simulink model "Verification"  (R2012b)
settings: Solver=FixedStepDiscrete  StartTime=0.0  StopTime=500  FixedStep=0.1  RelTol=1e-3
values from neighbouring files (symbols this model uses):
  high_safety_margin_s = 3.0    (= 3)    [constants.m]
  low_safety_margin_s = 3.0    (= 3)    [constants.m]
  tank1_cross_section_area_m2 = 1    [constants.m]
  tank1_max_vol_m3 = 7    [constants.m]
  tank1_safety_hi_ht_m = 5.0    (= 5)    [constants.m]
  tank1_safety_lo_ht_m = 2.0    (= 2)    [constants.m]
  tank2_cross_section_area_m2 = 2    [constants.m]
  tank2_max_vol_m3 = 8    [constants.m]
  tank2_safety_hi_ht_m = 3.0    (= 3)    [constants.m]
  time_increment_s = 0.1    [constants.m]
libraries: sldvlib x8
settings Model: Creator=Kerianne  LastModifiedBy=Kerianne
settings OptimizationCC: InlineParams=on

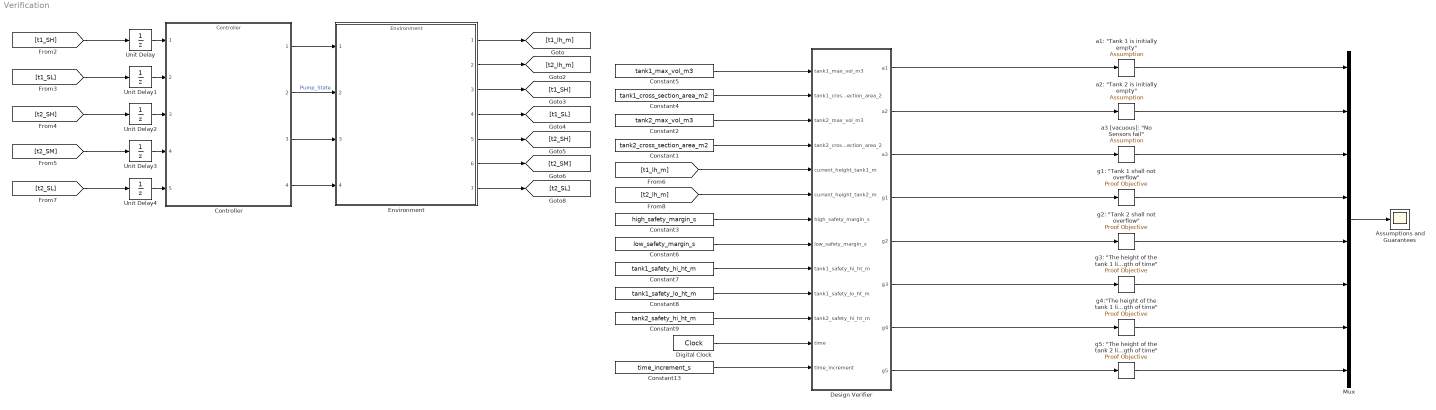
== system Verification ==
  " a2: \"Tank 2 is initially empty\" " : sldvlib/Objectives and Constraints/Assumption  enabled=on  customAVTBlockType=Assumption  intervals=true  initial=off  dispValues=on  outEnabled=on
      settings: AttributesFormatString=%<intervals>
  Assumptions and Guarantees : Scope
      settings: ShowLegends=on  TimeRange=500  YMin=0  YMax=2
  Constant1 : Constant  Value=tank2_cross_section_area_m2
  Constant13 : Constant  Value=time_increment_s
  Constant2 : Constant  Value=tank2_max_vol_m3
  Constant3 : Constant  Value=high_safety_margin_s
  Constant4 : Constant  Value=tank1_cross_section_area_m2
  Constant5 : Constant  Value=tank1_max_vol_m3
  Constant6 : Constant  Value=low_safety_margin_s
  Constant7 : Constant  Value=tank1_safety_hi_ht_m
  Constant8 : Constant  Value=tank1_safety_lo_ht_m
  Constant9 : Constant  Value=tank2_safety_hi_ht_m
  Controller : ModelReference  ModelNameDialog=Controller  SimulationMode=Normal  ModelReferenceVersion=1.19  CopyOfModelName=Controller  DefaultDataLogging=on
  Design Verifier : MATLAB Function  TreatAsAtomicUnit=on
  Digital Clock : DigitalClock  SampleTime=0.1
  Environment : ModelReference  ModelNameDialog=Environment  SimulationMode=Normal  ModelReferenceVersion=1.47  CopyOfModelName=Environment  DefaultDataLogging=on
  Mux : Mux  Inputs=8
  Unit Delay{,1..4} (5 alike) : UnitDelay  SampleTime=-1
  "a1: \"Tank 1 is initially empty\" " : sldvlib/Objectives and Constraints/Assumption  enabled=on  customAVTBlockType=Assumption  intervals=true  initial=off  dispValues=on  outEnabled=on
      settings: AttributesFormatString=%<intervals>
  "a3 [vacuous]: \"No Sensors fail\" " : sldvlib/Objectives and Constraints/Assumption  enabled=on  customAVTBlockType=Assumption  intervals=true  initial=off  dispValues=on  outEnabled=on
      settings: AttributesFormatString=%<intervals>
  "g1: \"Tank 1 shall not overflow\"" : sldvlib/Objectives and Constraints/Proof Objective  enabled=on  customAVTBlockType=Proof Objective  intervals=true  dispValues=on  outEnabled=on  enableStopSim=off
      settings: AttributesFormatString=%<intervals>
  "g2: \"Tank 2 shall not overflow\"" : sldvlib/Objectives and Constraints/Proof Objective  enabled=on  customAVTBlockType=Proof Objective  intervals=true  dispValues=on  outEnabled=on  enableStopSim=off
      settings: AttributesFormatString=%<intervals>
  "g3: \"The height of the tank 1 liquid shall not be over the tank 1 high safety level for more than the specified length of time\"" : sldvlib/Objectives and Constraints/Proof Objective  enabled=on  customAVTBlockType=Proof Objective  intervals=true  dispValues=on  outEnabled=on  enableStopSim=off
      settings: AttributesFormatString=%<intervals>
  "g4:\"The height of the tank 1 liquid shall not be lower than the tank 1 low safety level (once it has already crossed it) for more than the specified length of time\"" : sldvlib/Objectives and Constraints/Proof Objective  enabled=on  customAVTBlockType=Proof Objective  intervals=true  dispValues=on  outEnabled=on  enableStopSim=off
      settings: AttributesFormatString=%<intervals>
  "g5: \"The height of the tank 2 liquid shall not be over the tank 2 high safety level for more than the specified length of time\"" : sldvlib/Objectives and Constraints/Proof Objective  enabled=on  customAVTBlockType=Proof Objective  intervals=true  dispValues=on  outEnabled=on  enableStopSim=off
      settings: AttributesFormatString=%<intervals>
  wires:
  Design Verifier/1(a1) -> "a1: \"Tank 1 is initially empty\" "/1
  Digital Clock/1 -> Design Verifier/12(time)
  [t1_lh_m] -> Design Verifier/5(current_height_tank1_m)
  [t2_lh_m] -> Design Verifier/6(current_height_tank2_m)
  Design Verifier/2(a2) -> " a2: \"Tank 2 is initially empty\" "/1
  Mux/1 -> Assumptions and Guarantees/1
  Design Verifier/3(a3) -> "a3 [vacuous]: \"No Sensors fail\" "/1
  Design Verifier/4(g1) -> "g1: \"Tank 1 shall not overflow\""/1
  "g1: \"Tank 1 shall not overflow\""/1 -> Mux/4
  Design Verifier/5(g2) -> "g2: \"Tank 2 shall not overflow\""/1
  "g2: \"Tank 2 shall not overflow\""/1 -> Mux/5
  Design Verifier/8(g5) -> "g5: \"The height of the tank 2 liquid shall not be over the tank 2 high safety level for more than the specified length of time\""/1
  Design Verifier/7(g4) -> "g4:\"The height of the tank 1 liquid shall not be lower than the tank 1 low safety level (once it has already crossed it) for more than the specified length of time\""/1
  Design Verifier/6(g3) -> "g3: \"The height of the tank 1 liquid shall not be over the tank 1 high safety level for more than the specified length of time\""/1
  "g3: \"The height of the tank 1 liquid shall not be over the tank 1 high safety level for more than the specified length of time\""/1 -> Mux/6
  "g4:\"The height of the tank 1 liquid shall not be lower than the tank 1 low safety level (once it has already crossed it) for more than the specified length of time\""/1 -> Mux/7
  "g5: \"The height of the tank 2 liquid shall not be over the tank 2 high safety level for more than the specified length of time\""/1 -> Mux/8
  Constant13/1 -> Design Verifier/13(time_increment)
  Constant5/1 -> Design Verifier/1(tank1_max_vol_m3)
  Constant4/1 -> Design Verifier/2(tank1_cross_section_area_2)
  Constant2/1 -> Design Verifier/3(tank2_max_vol_m3)
  Constant1/1 -> Design Verifier/4(tank2_cross_section_area_2)
  Constant6/1 -> Design Verifier/8(low_safety_margin_s)
  Constant3/1 -> Design Verifier/7(high_safety_margin_s)
  Controller/1 -> Environment/1
  Controller/2 -> Environment/2  "Pump_State"
  Controller/3 -> Environment/3
  Controller/4 -> Environment/4
  [t1_SL] -> Unit Delay1/1
  [t2_SM] -> Unit Delay3/1
  [t1_SH] -> Unit Delay/1
  [t2_SH] -> Unit Delay2/1
  [t2_SL] -> Unit Delay4/1
  Environment/7 -> [t2_SL]
  Environment/6 -> [t2_SM]
  Environment/5 -> [t2_SH]
  Environment/4 -> [t1_SL]
  Environment/3 -> [t1_SH]
  Environment/2 -> [t2_lh_m]
  Environment/1 -> [t1_lh_m]
  Unit Delay/1 -> Controller/1
  Unit Delay1/1 -> Controller/2
  Unit Delay2/1 -> Controller/3
  Unit Delay3/1 -> Controller/4
  Unit Delay4/1 -> Controller/5
  Constant9/1 -> Design Verifier/11(tank2_safety_hi_ht_m)
  Constant8/1 -> Design Verifier/10(tank1_safety_lo_ht_m)
  Constant7/1 -> Design Verifier/9(tank1_safety_hi_ht_m)
  "a1: \"Tank 1 is initially empty\" "/1 -> Mux/1
  " a2: \"Tank 2 is initially empty\" "/1 -> Mux/2
  "a3 [vacuous]: \"No Sensors fail\" "/1 -> Mux/3

== matlab function Verification/Design Verifier ==
  data: tank1_max_vol_m3 input; a1 output; tank1_cross_section_area_2 input; tank2_max_vol_m3 input; tank2_cross_section_area_2 input; current_height_tank1_m input; current_height_tank2_m input; high_safety_margin_s input; low_safety_margin_s input; tank1_safety_hi_ht_m input; tank1_safety_lo_ht_m input; tank2_safety_hi_ht_m input; time input; time_increment input; a2 output; a3 output; g1 output; g2 output; g3 output; g4 output; g5 output
function [a1,a2,a3,g1,g2, g3, g4, g5] =...
    verification_condition(tank1_max_vol_m3, tank1_cross_section_area_2,...
    tank2_max_vol_m3,tank2_cross_section_area_2, current_height_tank1_m,...
    current_height_tank2_m, high_safety_margin_s,...
    low_safety_margin_s, tank1_safety_hi_ht_m, tank1_safety_lo_ht_m, ...
    tank2_safety_hi_ht_m,time, time_increment)
% Updated 3/6/2015 

tank1_height_m = tank1_max_vol_m3/tank1_cross_section_area_2;
tank2_height_m = tank2_max_vol_m3/tank2_cross_section_area_2;

persistent tank1_high_safety_timer
if isempty(tank1_high_safety_timer)
    tank1_high_safety_timer = 0;
elseif current_height_tank1_m > tank1_safety_hi_ht_m
    tank1_high_safety_timer = tank1_high_safety_timer + time_increment;
else
    tank1_high_safety_timer = 0;
end
persistent tank2_high_safety_timer
if isempty(tank2_high_safety_timer)
    tank2_high_safety_timer = 0;
elseif current_height_tank2_m > tank2_safety_hi_ht_m
    tank2_high_safety_timer = tank2_high_safety_timer + time_increment;
else
    tank2_high_safety_timer = 0;
end
persistent tank1_low_safety_timer
if isempty(tank1_low_safety_timer)
    tank1_low_safety_timer = 0;
elseif current_height_tank1_m < tank1_safety_lo_ht_m
    tank1_low_safety_timer = tank1_low_safety_timer + time_increment;
else
    tank1_low_safety_timer = 0;
end
persistent init_counter
if isempty(init_counter)
    init_counter = 0;
elseif current_height_tank1_m > tank1_safety_lo_ht_m
    init_counter = 1;
end

%%%%%%%%%%%%%%%%%%%%%%%%%%%%%%%%%%%%%%%%%%%%%%%%%%%%%%%%%%%%%%%%%%%%%%%%%
% Assumptions
% assume "Tank 1 shall initially be empty"
a1 = Tank_init_Empty(current_height_tank1_m, time);
% assume "Tank 2 shall initially be empty"
a2 = Tank_init_Empty(current_height_tank2_m, time);
% assume "No sensors fail":
a3 = true;

%%%%%%%%%%%%%%%%%%%%%%%%%%%%%%%%%%%%%%%%%%%%%%%%%%%%%%%%%%%%%%%%%%%%%%%%%
% Guarantees


% g1 guarantee "Tank 1 shall not overflow"
g1 = tank1_height_m >= current_height_tank1_m;

%  g2 guarantee "Tank 2 shall not overflow"
g2 = tank2_height_m >= current_height_tank2_m;

% g3 guarantee "The height of the tank 1 liquid shall not be over the tank 
% 1 high safety level for more than the specified length of time"
g3 = ((tank1_high_safety_timer < high_safety_margin_s) && ...
    (current_height_tank1_m < tank1_safety_hi_ht_m));
 
% g4 guarantee "The height of the tank 1 liquid shall not be lower than the 
% tank 1 low safety level (once it has already crossed it) for more than 
% the specified length of time"
g4 = ((tank1_low_safety_timer < low_safety_margin_s) && ...
    (current_height_tank1_m > tank1_safety_hi_ht_m)) | init_counter == 0;

% g5 guarantee "The height of the tank 2 liquid shall not be over the tank 
% 2 high safety level for more than the specified length of time":
g5 = ((tank2_high_safety_timer < high_safety_margin_s) && ...
    (current_height_tank2_m < tank2_safety_hi_ht_m));




% Called Functions
function c = implies(a,b)      
     c = ((not (a)) || b);
% a1 - a2
function result = Tank_init_Empty(current_height_tank_m, time) 
    UnderThisCondition = (time == 0.0);
    ResultShouldBe = (current_height_tank_m == 0.0);
    result = implies(UnderThisCondition, ResultShouldBe);
